simulink model "StepResponse_sim"  (R2017a)
settings: Solver=FixedStepAuto  StartTime=0.0  StopTime=Endtime  FixedStep=0.1  RelTol=1e-3
undefined symbols (not defined in the file): Humusoft, MF644, Ts
libraries: sldrtlib x5
settings Model: Creator=CSE2017  LastModifiedBy=CSE2017

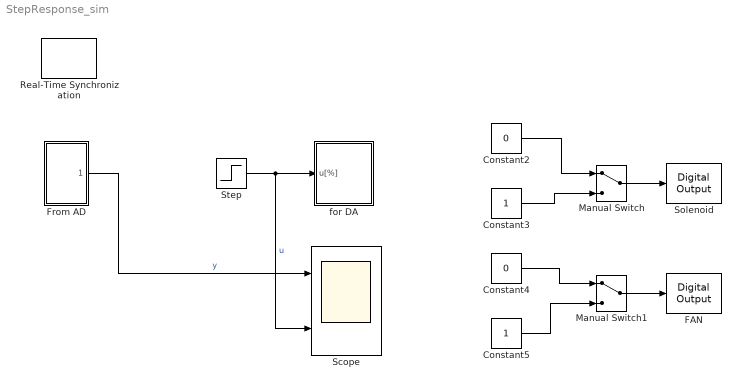
== system StepResponse_sim ==
  Constant2 : Constant  Value=0
  Constant3 : Constant
  Constant4 : Constant  Value=0
  Constant5 : Constant
  FAN : sldrtlib/Digital Output  SampleTime=Ts  MaxMissedTicks=10  ShowMissedTicks=off  YieldWhenWaiting=off  DrvName=Humusoft/MF644  DrvAddress=4294967295  DrvOptions=0  Channels=2  BitMode=1  InitialValue=0  FinalValue=0
      settings: AttributesFormatString=Humusoft\nMF644 [auto]  SourceProductName=Simulink Desktop Real-Time  SourceProductBaseCode=WT
  From AD : Subsystem
  Manual Switch : ManualSwitch
  Manual Switch1 : ManualSwitch
  Real-Time Synchronization : sldrtlib/Real-Time Synchronization  SampleTime=Ts  MaxMissedTicks=10  ShowMissedTicks=off  YieldWhenWaiting=off
  Scope : Scope  NumInputPorts=2
  Solenoid : sldrtlib/Digital Output  SampleTime=Ts  MaxMissedTicks=10  ShowMissedTicks=off  YieldWhenWaiting=off  DrvName=Humusoft/MF644  DrvAddress=4294967295  DrvOptions=0  Channels=1  BitMode=1  InitialValue=0  FinalValue=0
      settings: AttributesFormatString=Humusoft\nMF644 [auto]  SourceProductName=Simulink Desktop Real-Time  SourceProductBaseCode=WT
  Step : Step  Time=10  After=30  SampleTime=0
  for DA : Subsystem
  wires:
  Step/1 -> Scope/2, for DA/1(u[%])  "u"
  Constant2/1 -> Manual Switch/1
  Constant3/1 -> Manual Switch/2
  Constant4/1 -> Manual Switch1/1
  Constant5/1 -> Manual Switch1/2
  Manual Switch1/1 -> FAN/1
  Manual Switch/1 -> Solenoid/1
  From AD/1(y[deg.]) -> Scope/1  "y"

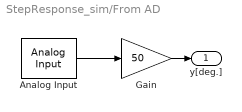
== system StepResponse_sim/From AD ==
  Analog Input : sldrtlib/Analog Input  SampleTime=Ts  MaxMissedTicks=10  ShowMissedTicks=off  YieldWhenWaiting=off  DrvName=Humusoft/MF644  DrvAddress=4294967295  DrvOptions=0  Channels=1  RangeMode=1  VoltRange=1  DataType=1
      settings: AttributesFormatString=Humusoft\nMF644 [auto]  SourceProductName=Simulink Desktop Real-Time
  Gain : Gain  Gain=50
  y[deg.] : Outport
  wires:
  Gain/1 -> y[deg.]/1
  Analog Input/1 -> Gain/1

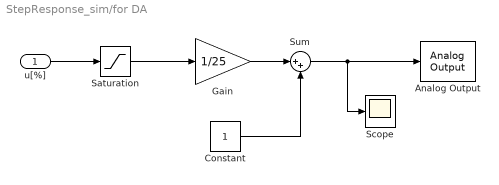
== system StepResponse_sim/for DA ==
  u[%] : Inport
  "Analog Output " : sldrtlib/Analog Output  SampleTime=Ts  MaxMissedTicks=10  ShowMissedTicks=off  YieldWhenWaiting=off  DrvName=Humusoft/MF644  DrvAddress=4294967295  DrvOptions=0  Channels=1  RangeMode=1  VoltRange=1  InitialValue=1  FinalValue=1
      settings: AttributesFormatString=Humusoft\nMF644 [auto]  SourceProductName=Simulink Desktop Real-Time
  Constant : Constant
  Gain : Gain  Gain=1/25
  Saturation : Saturate  UpperLimit=100  LowerLimit=0
  Scope : Scope
  Sum : Sum  Inputs=|++
  wires:
  Gain/1 -> Sum/1
  u[%]/1 -> Saturation/1
  Sum/1 -> Scope/1, "Analog Output "/1
  Constant/1 -> Sum/2
  Saturation/1 -> Gain/1
